simulink model "PMSM_MTPA_FOC"  (R2022a)
settings: Solver=VariableStepAuto  StartTime=0.0  StopTime=1  MaxStep=1e-4  MinStep=1e-6  RelTol=1e-3
InitFcn:
  | Ts = 1e-5;
  | Tpwm = 1e-4;
  | Udc = 650;
  | 
  | R = 0.077;
  | Ld = 1.5e-3;
  | Lq = 3e-3;
  | Pn = 4;
  | Flux = 0.11;
undefined symbols (not defined in the file or in its folder): DiscIntNeverNeededParam
libraries: spsDCVoltageSourceLib x1, spsPermanentMagnetSynchronousMachineLib x1, simulink x1, spsUniversalBridgeLib x1, spsVoltageMeasurementLib x1, spspowerguiLib x1
settings Model: Creator=LXP  LastModifiedBy=LXP
settings DataIOCC: SaveFormat=StructureWithTime  ReturnWorkspaceOutputsName=mtpaout

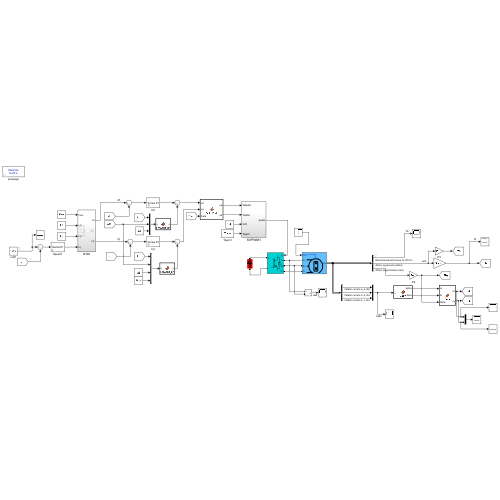
[thumbnail: Simulink's stored preview of the top-level diagram]
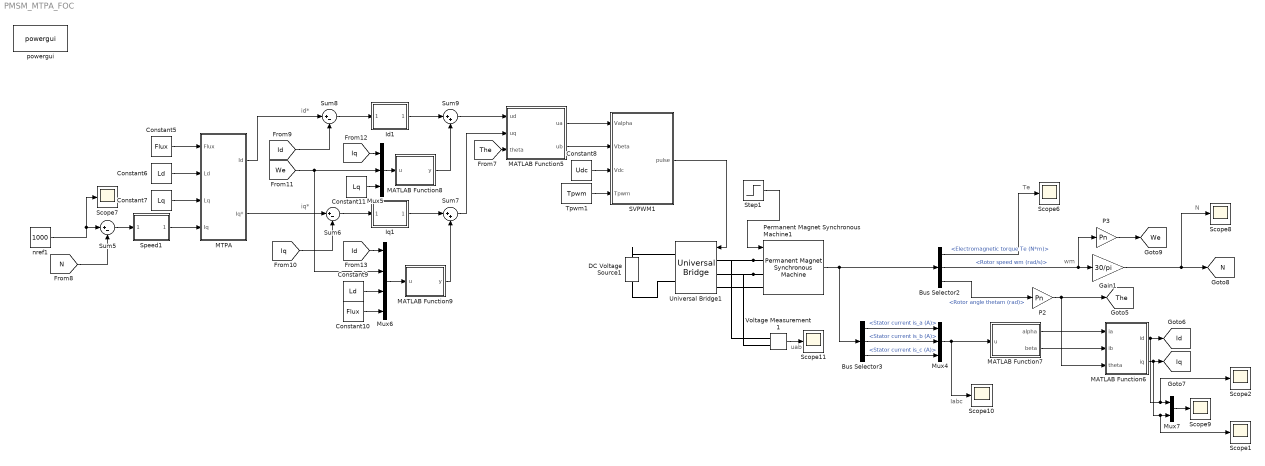
== system PMSM_MTPA_FOC ==
  note: Te
  note: wm
  note: iq*
  note: Iabc
  note: uab
  note: N
  note: id*
  Bus Selector2 : BusSelector  OutputSignals=Electromagnetic torque Te (N*m),Rotor speed wm (rad/s),Rotor angle thetam (rad)
  Bus Selector3 : BusSelector  OutputSignals=Stator current is_a (A),Stator current is_b (A),Stator current is_c (A)
  Constant10 : Constant  Value=Flux
  Constant11 : Constant  Value=Lq
  Constant5 : Constant  Value=Flux
  Constant6 : Constant  Value=Ld
  Constant7 : Constant  Value=Lq
  Constant8 : Constant  Value=Udc
  Constant9 : Constant  Value=Ld
  DC Voltage Source1 : spsDCVoltageSourceLib/DC Voltage Source  Amplitude=Udc  Measurements=None
  Gain1 : Gain  Gain=30/pi
  Id1 : Subsystem  mask{Ka=4.71, Kb=51.33, Ts=Ts, I_limit=[-375 375], PI_limit=[-375 375]}
      mask prompts: Ka "Proportional gain(Ka)："; Kb "Integral gain(Kb)："; Ts "Sampling time(Ts)："; I_limit "I Output limit:[ Imin Imax ]"; PI_limit "PI Output limit:[ Lowerlimit Upperlimit ]"
      mask init:
      | Imin=I_limit(1);
      | Imax=I_limit(2);
      | 
      | Lowerlimit = PI_limit(1);
      | Upperlimit = PI_limit(2);
      | power_initmask();
      mask DialogControl ParameterGroupVar Prompt: 参数
      mask Display: disp('Series PI');
  Iq1 : Subsystem  mask{Ka=9.43, Kb=25.67, Ts=Ts, I_limit=[-375 375], PI_limit=[-375 375]}
      mask prompts: Ka "Proportional gain(Ka)："; Kb "Integral gain(Kb)："; Ts "Sampling time(Ts)："; I_limit "I Output limit:[ Imin Imax ]"; PI_limit "PI Output limit:[ Lowerlimit Upperlimit ]"
      mask init:
      | Imin=I_limit(1);
      | Imax=I_limit(2);
      | 
      | Lowerlimit = PI_limit(1);
      | Upperlimit = PI_limit(2);
      | power_initmask();
      mask DialogControl ParameterGroupVar Prompt: 参数
      mask Display: disp('Series PI');
  MATLAB Function5 : MATLAB Function  TreatAsAtomicUnit=on
  MATLAB Function6 : MATLAB Function  TreatAsAtomicUnit=on
  MATLAB Function7 : MATLAB Function  TreatAsAtomicUnit=on
  MATLAB Function8 : MATLAB Function  TreatAsAtomicUnit=on
  MATLAB Function9 : MATLAB Function  TreatAsAtomicUnit=on
  MTPA : Subsystem
  Mux4 : Mux  Inputs=3
  Mux5 : Mux  Inputs=3
  Mux6 : Mux
  Mux7 : Mux  Inputs=2
  P2 : Gain  Gain=Pn
  P3 : Gain  Gain=Pn
  Permanent Magnet Synchronous Machine1 : spsPermanentMagnetSynchronousMachineLib/Permanent Magnet Synchronous Machine  NbPhases=3  FluxDistribution=Sinusoidal  RotorType=Salient-pole  MechanicalLoad=Torque Tm  PresetModel=No  ShowDetailedParameters=on  MeasurementBus=off  Resistance=0.077  Inductance=8.5e-3  dqInductances=[1.5e-3,3e-3]  La=0.000395  MachineConstant=Flux linkage established by magnets (V.s)  Flux=0.11  VoltageCst=79.8072  TorqueCst=0.66  Flat=120  Mechanical=[0.1 0.0004924 4 0]  PolePairs=4  InitialConditions=[0,0, 0,0]  InitialConditions5ph=[0 0 0 0 0 0]  RefAngle=Aligned with phase A axis (original Park)  IterativeDiscreteModel=Trapezoidal non iterative  TsBlock=-1  TsPowergui=0
  SVPWM1 : Subsystem
  Scope{1..2,6..11} (8 alike) : Scope
  Speed1 : Subsystem  mask{Ka=7.86, Kb=31.43, Ts=Ts, I_limit=[-236 236], PI_limit=[-236 236]}
      mask prompts: Ka "Proportional gain(Ka)："; Kb "Integral gain(Kb)："; Ts "Sampling time(Ts)："; I_limit "I Output limit:[ Imin Imax ]"; PI_limit "PI Output limit:[ Lowerlimit Upperlimit ]"
      mask init:
      | Imin=I_limit(1);
      | Imax=I_limit(2);
      | 
      | Lowerlimit = PI_limit(1);
      | Upperlimit = PI_limit(2);
      | power_initmask();
      mask DialogControl ParameterGroupVar Prompt: 参数
      mask Display: disp('Series PI');
  Step1 : Step  Time=0.5  After=100  SampleTime=0
  Sum5 : Sum  Inputs=|+-
  Sum6 : Sum  Inputs=|+-
  Sum7 : Sum  Inputs=|++
  Sum8 : Sum  Inputs=|+-
  Sum9 : Sum  Inputs=|++
  Tpwm1 : Constant  Value=Tpwm
  Universal Bridge1 : spsUniversalBridgeLib/Universal Bridge  Arms=3  SnubberResistance=1e5  SnubberCapacitance=inf  Device=IGBT / Diodes  Ron=1e-3  Lon=0  ForwardVoltages="[  0  0  ]"  ForwardVoltage=0  GTOparameters=[ 10e-6 , 20e-6 ]  IGBTparameters=[ 1e-6 , 2e-6 ]  Measurements=None  Measurements_2=None  converterType=Rectifier
  Voltage Measurement1 : spsVoltageMeasurementLib/Voltage Measurement  PhasorSimulation=off  OutputType=Complex  PSBequivalent=0
  nref1 : Constant  Value=1000  SampleTime=1e-5
  powergui : spspowerguiLib/powergui  Priority=1  SimulationMode=Discrete  SampleTime=1e-5  frequency=60  Iterations=50  frequencyindice=0  Pbase=100e6  ErrMax=1e-4  UnitsV=kV  UnitsW=MW  buscounter=0  FunctionMessages=off  echomessages=off  EnableUseOfTLC=off  CurrentSourceSwitches=off  DisableSnubberDevices=off  DisableRonSwitches=off  DisableVfSwitches=off  DisplayEquations=off  AutomaticDiscreteSolvers=off  SolverType=Tustin/Backward Euler (TBE)  Interpol=off  ExternalGateDelay=off  methode=off  Ts=100  x0status=blocks  SPID=on  SwTol=0  HookPort=off  NonlinearTolerance=1e-4  nMaxIteration=100  ContinueOnMaxIteration=off  RestoreLinks=warning  ResistiveCurrentMeasurement=off  Frange=[0:2:500]  Ylog=off  Xlog=on  ShowGrid=off  save=off  variable=ZData  structure=0  ZoomFFT=off  StartTime=0.0  cycles=1  DisplayStyle=1  fundamental=60  FreqAxis=off  MaxFrequency=1000  frequencyindicesteady=1  RmsSteady=1  display=off
  tag scope: Id=global, Iq=global, N=global, The=global, We=global
  wires:
  Gain1/1 -> Scope8/1, [N]
  [N] -> Sum5/2
  Bus Selector2/2 -> P3/1, Gain1/1  "<Rotor speed wm (rad/s)>"
  P3/1 -> [We]
  Constant11/1 -> Mux5/3
  Id1/1(Output) -> Sum9/1
  Voltage Measurement1/1 -> Scope11/1
  Mux5/1 -> MATLAB Function8/1(u)
  Constant8/1 -> SVPWM1/3(Vdc)
  Constant10/1 -> Mux6/4
  Bus Selector3/1 -> Mux4/1  "<Stator current is_a (A)>"
  Sum5/1 -> Speed1/1(Error)
  Mux6/1 -> MATLAB Function9/1(u)
  MATLAB Function5/2(ub) -> SVPWM1/2(Vbeta)
  Sum7/1 -> MATLAB Function5/2(uq)
  MATLAB Function5/1(ua) -> SVPWM1/1(Valpha)
  Sum8/1 -> Id1/1(Error)
  Sum9/1 -> MATLAB Function5/1(ud)
  Constant9/1 -> Mux6/3
  [Id] -> Sum8/2
  Bus Selector2/1 -> Scope6/1  "<Electromagnetic torque Te (N*m)>"
  Permanent Magnet Synchronous Machine1/1 -> Bus Selector3/1, Bus Selector2/1
  MATLAB Function7/1(alpha) -> MATLAB Function6/1(ia)
  [Iq] -> Sum6/2
  Sum6/1 -> Iq1/1(Error)
  [Iq] -> Mux5/1
  [We] -> Mux5/2, Mux6/2
  [The] -> MATLAB Function5/3(theta)
  Bus Selector2/3 -> P2/1  "<Rotor angle thetam (rad)>"
  Bus Selector3/3 -> Mux4/3  "<Stator current is_c (A)>"
  P2/1 -> MATLAB Function6/3(theta), [The]
  SVPWM1/1(pulse) -> Universal Bridge1/1
  Speed1/1(Output) -> MTPA/4(Iq)
  Iq1/1(Output) -> Sum7/1
  MATLAB Function6/2(iq) -> Scope1/1, Mux7/2, [Iq]
  Step1/1 -> Permanent Magnet Synchronous Machine1/1
  nref1/1 -> Sum5/1, Scope7/1
  Tpwm1/1 -> SVPWM1/4(Tpwm)
  MATLAB Function9/1(y) -> Sum7/2
  Bus Selector3/2 -> Mux4/2  "<Stator current is_b (A)>"
  MATLAB Function6/1(id) -> Scope2/1, Mux7/1, [Id]
  [Id] -> Mux6/1
  Mux7/1 -> Scope9/1
  MTPA/1(Id) -> Sum8/1
  Constant5/1 -> MTPA/1(Flux)
  MATLAB Function7/2(beta) -> MATLAB Function6/2(ib)
  Constant7/1 -> MTPA/3(Lq)
  MATLAB Function8/1(y) -> Sum9/2
  MTPA/2(Iq*) -> Sum6/1
  Constant6/1 -> MTPA/2(Ld)
  Mux4/1 -> MATLAB Function7/1(u), Scope10/1
  connections:
  Permanent Magnet Synchronous Machine1/LConn1 -- Universal Bridge1/LConn1 -- Voltage Measurement1/LConn1
  Permanent Magnet Synchronous Machine1/LConn2 -- Universal Bridge1/LConn2 -- Voltage Measurement1/LConn2
  Universal Bridge1/RConn2 -- DC Voltage Source1/LConn1
  DC Voltage Source1/RConn1 -- Universal Bridge1/RConn1
  Universal Bridge1/LConn3 -- Permanent Magnet Synchronous Machine1/LConn3

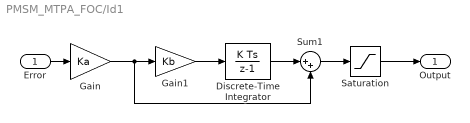
== system PMSM_MTPA_FOC/Id1 ==
  Error : Inport
  Discrete-Time Integrator : DiscreteIntegrator  SampleTime=Ts  LimitOutput=on  UpperSaturationLimit=Imax  LowerSaturationLimit=Imin  ICPrevOutput=DiscIntNeverNeededParam  ICPrevScaledInput=DiscIntNeverNeededParam
  Gain : Gain  Gain=Ka
  Gain1 : Gain  Gain=Kb
  Saturation : Saturate  UpperLimit=Upperlimit  LowerLimit=Lowerlimit
  Sum1 : Sum  Inputs=|++
  Output : Outport
  wires:
  Gain/1 -> Sum1/2, Gain1/1
  Gain1/1 -> Discrete-Time Integrator/1
  Error/1 -> Gain/1
  Discrete-Time Integrator/1 -> Sum1/1
  Sum1/1 -> Saturation/1
  Saturation/1 -> Output/1

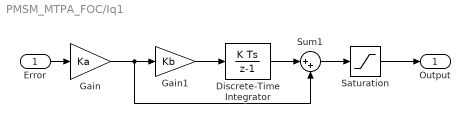
== system PMSM_MTPA_FOC/Iq1 ==
  Error : Inport
  Discrete-Time Integrator : DiscreteIntegrator  SampleTime=Ts  LimitOutput=on  UpperSaturationLimit=Imax  LowerSaturationLimit=Imin  ICPrevOutput=DiscIntNeverNeededParam  ICPrevScaledInput=DiscIntNeverNeededParam
  Gain : Gain  Gain=Ka
  Gain1 : Gain  Gain=Kb
  Saturation : Saturate  UpperLimit=Upperlimit  LowerLimit=Lowerlimit
  Sum1 : Sum  Inputs=|++
  Output : Outport
  wires:
  Gain/1 -> Sum1/2, Gain1/1
  Gain1/1 -> Discrete-Time Integrator/1
  Error/1 -> Gain/1
  Discrete-Time Integrator/1 -> Sum1/1
  Sum1/1 -> Saturation/1
  Saturation/1 -> Output/1

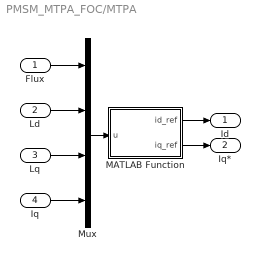
== system PMSM_MTPA_FOC/MTPA ==
  Flux : Inport
  Ld : Inport  Port=2
  Lq : Inport  Port=3
  Iq : Inport  Port=4
  MATLAB Function : MATLAB Function  TreatAsAtomicUnit=on
  Mux : Mux
  Id : Outport
  Iq* : Outport  Port=2
  wires:
  Flux/1 -> Mux/1
  Ld/1 -> Mux/2
  Lq/1 -> Mux/3
  Iq/1 -> Mux/4
  Mux/1 -> MATLAB Function/1(u)
  MATLAB Function/1(id_ref) -> Id/1
  MATLAB Function/2(iq_ref) -> Iq*/1

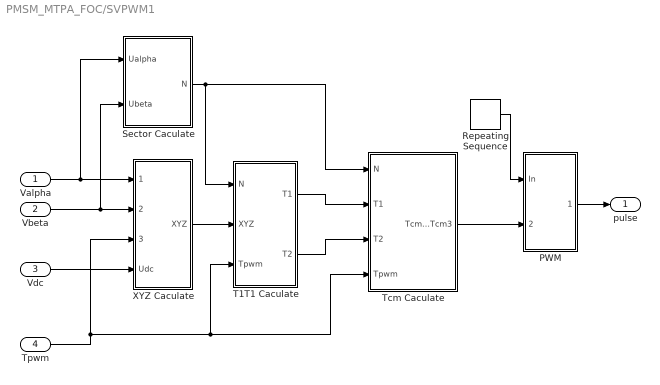
== system PMSM_MTPA_FOC/SVPWM1 ==
  Valpha : Inport
  Vbeta : Inport  Port=2
  Vdc : Inport  Port=3
  Tpwm : Inport  Port=4
  PWM : Subsystem
  Repeating Sequence : simulink/Sources/Repeating Sequence  rep_seq_t=[0 0.00005 0.0001]  rep_seq_y=[0 0.00005 0]
  Sector Caculate : Subsystem
  T1T1 Caculate : Subsystem
  Tcm Caculate : Subsystem
  XYZ Caculate : Subsystem
  pulse : Outport  VectorParamsAs1DForOutWhenUnconnected=off
  wires:
  PWM/1(PWM) -> pulse/1
  Repeating Sequence/1 -> PWM/1(In)
  Vbeta/1 -> XYZ Caculate/2(Ubeta), Sector Caculate/2(Ubeta)
  T1T1 Caculate/1(T1) -> Tcm Caculate/2(T1)
  Valpha/1 -> XYZ Caculate/1(Ualpha), Sector Caculate/1(Ualpha)
  T1T1 Caculate/2(T2) -> Tcm Caculate/3(T2)
  Sector Caculate/1("N ") -> Tcm Caculate/1(N), T1T1 Caculate/1(N)
  XYZ Caculate/1(XYZ) -> T1T1 Caculate/2(XYZ)
  Tpwm/1 -> XYZ Caculate/3(Tpwm), Tcm Caculate/4(Tpwm), T1T1 Caculate/3(Tpwm)
  Vdc/1 -> XYZ Caculate/4(Udc)
  Tcm Caculate/1(Tcm1 Tcm2 Tcm3) -> PWM/2(Tcm123)

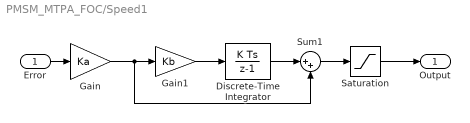
== system PMSM_MTPA_FOC/Speed1 ==
  Error : Inport
  Discrete-Time Integrator : DiscreteIntegrator  SampleTime=Ts  LimitOutput=on  UpperSaturationLimit=Imax  LowerSaturationLimit=Imin  ICPrevOutput=DiscIntNeverNeededParam  ICPrevScaledInput=DiscIntNeverNeededParam
  Gain : Gain  Gain=Ka
  Gain1 : Gain  Gain=Kb
  Saturation : Saturate  UpperLimit=Upperlimit  LowerLimit=Lowerlimit
  Sum1 : Sum  Inputs=|++
  Output : Outport
  wires:
  Gain/1 -> Sum1/2, Gain1/1
  Gain1/1 -> Discrete-Time Integrator/1
  Error/1 -> Gain/1
  Discrete-Time Integrator/1 -> Sum1/1
  Sum1/1 -> Saturation/1
  Saturation/1 -> Output/1

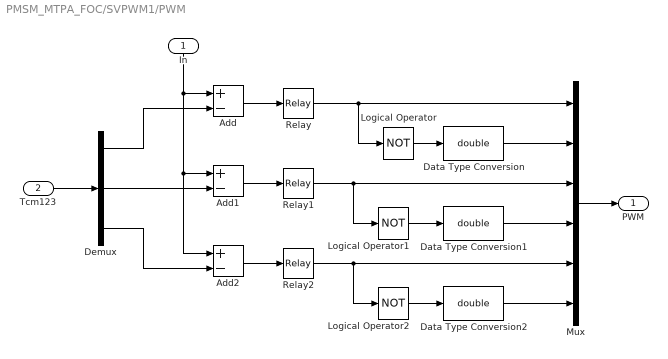
== system PMSM_MTPA_FOC/SVPWM1/PWM ==
  In : Inport
  Tcm123 : Inport  Port=2
  Add : Sum  Inputs=+-
  Add1 : Sum  Inputs=+-
  Add2 : Sum  Inputs=+-
  Data Type Conversion : DataTypeConversion  OutDataTypeStr=double  SaturateOnIntegerOverflow=off  RndMeth=Floor
  Data Type Conversion1 : DataTypeConversion  OutDataTypeStr=double  SaturateOnIntegerOverflow=off  RndMeth=Floor
  Data Type Conversion2 : DataTypeConversion  OutDataTypeStr=double  SaturateOnIntegerOverflow=off  RndMeth=Floor
  Demux : Demux  Outputs=3
  Logical Operator : Logic  Operator=NOT  AllPortsSameDT=off  OutDataTypeStr=boolean
  Logical Operator1 : Logic  Operator=NOT  AllPortsSameDT=off  OutDataTypeStr=boolean
  Logical Operator2 : Logic  Operator=NOT  AllPortsSameDT=off  OutDataTypeStr=boolean
  Mux : Mux  Inputs=6
  Relay : Relay  OffSwitchValue=-eps
  Relay1 : Relay  OffSwitchValue=-eps
  Relay2 : Relay  OffSwitchValue=-eps
  PWM : Outport  VectorParamsAs1DForOutWhenUnconnected=off
  wires:
  Demux/3 -> Add2/2
  Demux/2 -> Add1/2
  Demux/1 -> Add/2
  Relay2/1 -> Mux/5, Logical Operator2/1
  Relay1/1 -> Mux/3, Logical Operator1/1
  Relay/1 -> Logical Operator/1, Mux/1
  Mux/1 -> PWM/1
  Data Type Conversion/1 -> Mux/2
  Data Type Conversion1/1 -> Mux/4
  Data Type Conversion2/1 -> Mux/6
  Logical Operator2/1 -> Data Type Conversion2/1
  Logical Operator1/1 -> Data Type Conversion1/1
  Logical Operator/1 -> Data Type Conversion/1
  Add1/1 -> Relay1/1
  Add2/1 -> Relay2/1
  Add/1 -> Relay/1
  In/1 -> Add/1, Add2/1, Add1/1
  Tcm123/1 -> Demux/1

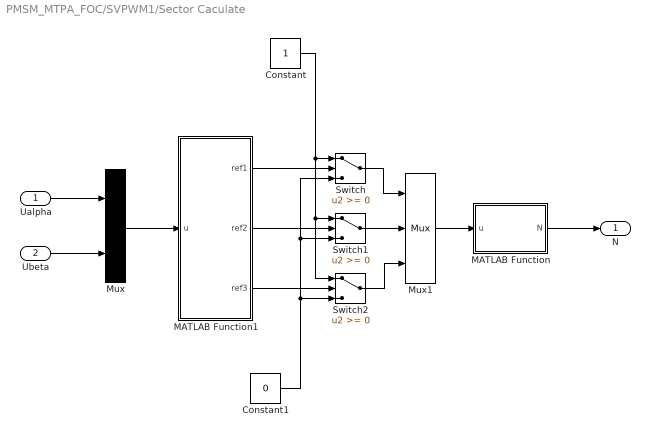
== system PMSM_MTPA_FOC/SVPWM1/Sector Caculate ==
  Ualpha : Inport
  Ubeta : Inport  Port=2
  Constant : Constant
  Constant1 : Constant  Value=0
  MATLAB Function : MATLAB Function  TreatAsAtomicUnit=on
  MATLAB Function1 : MATLAB Function  TreatAsAtomicUnit=on
  Mux : Mux  Inputs=2
  Mux1 : Mux  Inputs=3
  Switch : Switch  SaturateOnIntegerOverflow=off  InputSameDT=off
  Switch1 : Switch  SaturateOnIntegerOverflow=off  InputSameDT=off
  Switch2 : Switch  SaturateOnIntegerOverflow=off  InputSameDT=off
  "N " : Outport  VectorParamsAs1DForOutWhenUnconnected=off
  wires:
  Switch2/1 -> Mux1/3
  Switch/1 -> Mux1/1
  Ualpha/1 -> Mux/1
  Ubeta/1 -> Mux/2
  MATLAB Function1/1(ref1) -> Switch/2
  MATLAB Function1/2(ref2) -> Switch1/2
  MATLAB Function1/3(ref3) -> Switch2/2
  Constant/1 -> Switch/1, Switch2/1, Switch1/1
  Constant1/1 -> Switch/3, Switch1/3, Switch2/3
  Switch1/1 -> Mux1/2
  Mux1/1 -> MATLAB Function/1(u)
  MATLAB Function/1(N) -> "N "/1
  Mux/1 -> MATLAB Function1/1(u)

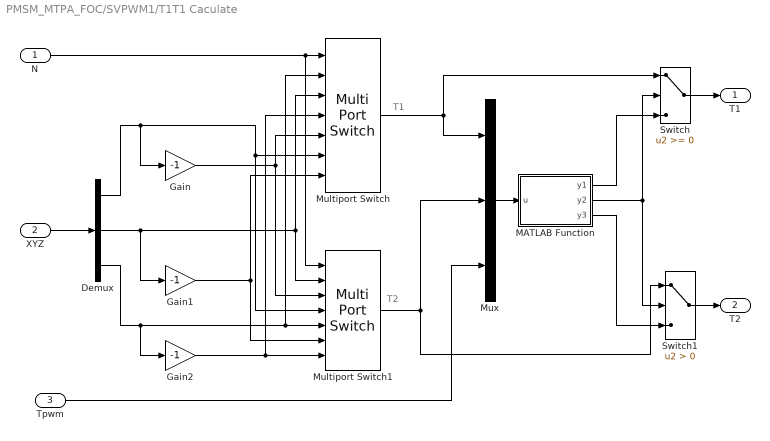
== system PMSM_MTPA_FOC/SVPWM1/T1T1 Caculate ==
  note: T1
  note: T2
  N : Inport
  XYZ : Inport  Port=2
  Tpwm : Inport  Port=3
  Demux : Demux  Outputs=3
  Gain : Gain  Gain=-1
  Gain1 : Gain  Gain=-1
  Gain2 : Gain  Gain=-1
  MATLAB Function : MATLAB Function  TreatAsAtomicUnit=on
  Multiport Switch : MultiPortSwitch  Inputs=6  SaturateOnIntegerOverflow=off  InputSameDT=off
  Multiport Switch1 : MultiPortSwitch  Inputs=6  SaturateOnIntegerOverflow=off  InputSameDT=off
  Mux : Mux  Inputs=3
  Switch : Switch  SaturateOnIntegerOverflow=off  InputSameDT=off
  Switch1 : Switch  Criteria=u2 > Threshold  SaturateOnIntegerOverflow=off  InputSameDT=off
  T1 : Outport  VectorParamsAs1DForOutWhenUnconnected=off
  T2 : Outport  Port=2  VectorParamsAs1DForOutWhenUnconnected=off
  wires:
  Tpwm/1 -> Mux/3
  XYZ/1 -> Demux/1
  Switch1/1 -> T2/1
  Switch/1 -> T1/1
  MATLAB Function/3(y3) -> Switch1/3
  MATLAB Function/1(y1) -> Switch/3
  MATLAB Function/2(y2) -> Switch/2, Switch1/2
  Mux/1 -> MATLAB Function/1(u)
  Multiport Switch/1 -> Switch/1, Mux/1
  Multiport Switch1/1 -> Switch1/1, Mux/2
  N/1 -> Multiport Switch/1, Multiport Switch1/1
  Demux/2 -> Multiport Switch/3, Multiport Switch1/2, Gain1/1
  Demux/3 -> Multiport Switch1/5, Multiport Switch/2, Gain2/1
  Demux/1 -> Multiport Switch/6, Multiport Switch1/4, Gain/1
  Gain/1 -> Multiport Switch1/3, Multiport Switch/5
  Gain2/1 -> Multiport Switch/4, Multiport Switch1/7
  Gain1/1 -> Multiport Switch1/6, Multiport Switch/7

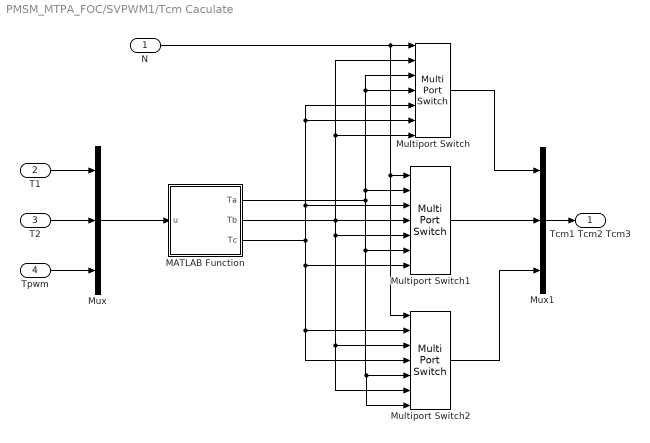
== system PMSM_MTPA_FOC/SVPWM1/Tcm Caculate ==
  N : Inport
  T1 : Inport  Port=2
  T2 : Inport  Port=3
  Tpwm : Inport  Port=4
  MATLAB Function : MATLAB Function  TreatAsAtomicUnit=on
  Multiport Switch : MultiPortSwitch  Inputs=6  SaturateOnIntegerOverflow=off  InputSameDT=off
  Multiport Switch1 : MultiPortSwitch  Inputs=6  SaturateOnIntegerOverflow=off  InputSameDT=off
  Multiport Switch2 : MultiPortSwitch  Inputs=6  SaturateOnIntegerOverflow=off  InputSameDT=off
  Mux : Mux  Inputs=3
  Mux1 : Mux  Inputs=3
  Tcm1 Tcm2 Tcm3 : Outport  VectorParamsAs1DForOutWhenUnconnected=off
  wires:
  Tpwm/1 -> Mux/3
  T2/1 -> Mux/2
  T1/1 -> Mux/1
  Multiport Switch2/1 -> Mux1/3
  Multiport Switch1/1 -> Mux1/2
  Multiport Switch/1 -> Mux1/1
  Mux1/1 -> Tcm1 Tcm2 Tcm3/1
  MATLAB Function/1(Ta) -> Multiport Switch/3, Multiport Switch/4, Multiport Switch1/2, Multiport Switch1/6, Multiport Switch2/5, Multiport Switch2/7
  MATLAB Function/2(Tb) -> Multiport Switch1/5, Multiport Switch2/3, Multiport Switch2/6, Multiport Switch1/4, Multiport Switch/7, Multiport Switch/2
  MATLAB Function/3(Tc) -> Multiport Switch2/2, Multiport Switch2/4, Multiport Switch1/7, Multiport Switch/5, Multiport Switch/6, Multiport Switch1/3
  N/1 -> Multiport Switch2/1, Multiport Switch1/1, Multiport Switch/1
  Mux/1 -> MATLAB Function/1(u)

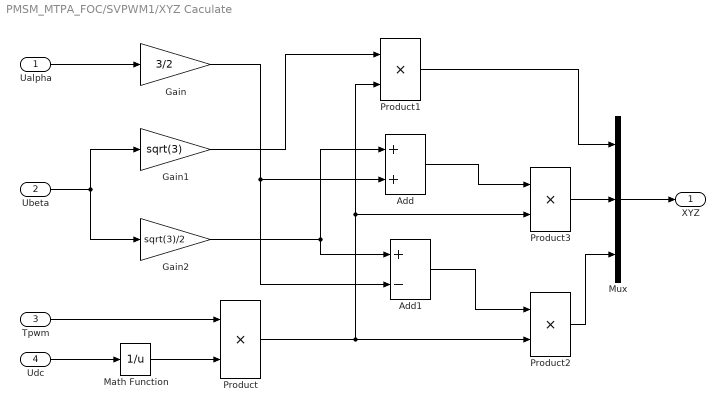
== system PMSM_MTPA_FOC/SVPWM1/XYZ Caculate ==
  Ualpha : Inport
  Ubeta : Inport  Port=2
  Tpwm : Inport  Port=3
  Udc : Inport  Port=4
  Add : Sum
  Add1 : Sum  Inputs=+-
  Gain : Gain  Gain=3/2
  Gain1 : Gain  Gain=sqrt(3)
  Gain2 : Gain  Gain=sqrt(3)/2
  Math Function : Math  Operator=reciprocal  SignedPower=on
  Mux : Mux  Inputs=3
  Product{,1..3} (4 alike) : Product  RndMeth=Zero
  XYZ : Outport  VectorParamsAs1DForOutWhenUnconnected=off
  wires:
  Mux/1 -> XYZ/1
  Product1/1 -> Mux/1
  Product3/1 -> Mux/2
  Product2/1 -> Mux/3
  Ualpha/1 -> Gain/1
  Ubeta/1 -> Gain2/1, Gain1/1
  Udc/1 -> Math Function/1
  Math Function/1 -> Product/2
  Tpwm/1 -> Product/1
  Gain1/1 -> Product1/1
  Product/1 -> Product2/2, Product1/2, Product3/2
  Gain/1 -> Add1/2, Add/2
  Gain2/1 -> Add/1, Add1/1
  Add1/1 -> Product2/1
  Add/1 -> Product3/1

== matlab function PMSM_MTPA_FOC/MTPA/MATLAB Function ==
  data: u input; id_ref output; iq_ref output
function [id_ref,iq_ref] = fcn(u)
    deltaL = u(2)-u(3);
    id_ref_den = (-u(1)+sqrt(u(1)^2 + 4*deltaL^2*u(4)^2));
    id_ref = id_ref_den/(2*deltaL);
    iq_ref = u(4);

== matlab function PMSM_MTPA_FOC/MATLAB Function5 ==
  data: ua output; ud input; uq input; theta input; ub output
function [ua,ub] =  Anti_Park(ud,uq,theta)

ua = cos(theta)*ud - sin(theta)*uq;
ub = sin(theta)*ud + cos(theta)*uq;

== matlab function PMSM_MTPA_FOC/MATLAB Function6 ==
  data: id output; ia input; ib input; theta input; iq output
function [id,iq] =  Park(ia,ib,theta)

id = cos(theta)*ia + sin(theta)*ib;
iq =-sin(theta)*ia + cos(theta)*ib;

== matlab function PMSM_MTPA_FOC/MATLAB Function7 ==
  data: u input; alpha output; beta output
function [alpha,beta] = Clark(u)
    alpha = (u(1)-0.5*(u(2)+u(3)))*2/3;
    beta = sqrt(3)/2*(u(2)-u(3))*2/3;

== matlab function PMSM_MTPA_FOC/MATLAB Function8 ==
  data: u input; y output
function y = Forward_ud(u)
Lq = u(3);
y = -Lq*u(1)*u(2);

== matlab function PMSM_MTPA_FOC/MATLAB Function9 ==
  data: u input; y output
function y = Forward_uq(u)
    Ld = u(3);
    Flux = u(4);
    y = u(2)*(Ld*u(1)+Flux);

== matlab function PMSM_MTPA_FOC/SVPWM1/Sector Caculate/MATLAB Function ==
  data: u input; N output
function N = Ngen(u)

    N = u(1) + 2*u(2) + 4*u(3);

== matlab function PMSM_MTPA_FOC/SVPWM1/Sector Caculate/MATLAB Function1 ==
  data: ref1 output; u input; ref2 output; ref3 output
function [ref1, ref2, ref3] = Vref(u)
    ref1 = u(2);
    ref2 = sqrt(3/4)*u(1) - 0.5*u(2);
    ref3 = -sqrt(3/4)*u(1) - 0.5*u(2);

== matlab function PMSM_MTPA_FOC/SVPWM1/T1T1 Caculate/MATLAB Function ==
  data: u input; y1 output; y2 output; y3 output
function [y1,y2,y3] = fcn(u)
    y1 = u(1)*u(3)/(u(1)+u(2));
    y2 = u(3)-u(2)-u(1);
    y3 = u(1)*u(3)/(u(1)+u(2));

== matlab function PMSM_MTPA_FOC/SVPWM1/Tcm Caculate/MATLAB Function ==
  data: u input; Ta output; Tb output; Tc output
function [Ta,Tb,Tc] = TimeCal(u)
    Ta = (u(3)-u(2)-u(1))/4;
    Tb = (u(3)+u(1)-u(2))/4;
    Tc = (u(3)+u(2)+u(1))/4;
